simulink model "exploration"  (R2019a)
settings: Solver=FixedStepAuto  StartTime=0.0  StopTime=inf  FixedStep=0.001  RelTol=1e-3  EnableMultiTasking=on
settings Model: ExtModeTrigDuration=2  Creator=Dell  LastModifiedBy=Apple
settings OptimizationCC: EnhancedBackFolding=on  PassReuseOutputArgsAs=Individual arguments  MaxStackSize=64  OptimizeBlockOrder=speed  DifferentSizesBufferReuse=on  OptimizationCustomize=off
settings DebuggingCC: ParameterTunabilityLossMsg=error
settings HardwareCC: ProdBitPerInt=16  ProdBitPerPointer=16  ProdBitPerSizeT=16  ProdBitPerPtrDiffT=16  ProdLargestAtomicFloat=None  ProdWordSize=8  ProdHWDeviceType=Atmel->AVR  UseEmbeddedCoderFeatures=off
settings SFSimCC: MATLABDynamicMemAlloc=off
settings RTWCC: SystemTargetFile=ert.tlc  HardwareBoard=Arduino Mega 2560  TLCOptions=-aInlineSetEventsForThisBaseRateFcn=TLC_FALSE -aSuppressMultiTaskScheduler=TLC_FALSE -aRateBasedStepFcn=1  TemplateMakefile=ert_default_tmf  GenerateReport=on  Toolchain=Arduino AVR  BuildConfiguration=Faster Runs  IncludeHyperlinkInReport=on  LaunchReport=on  GenerateTraceInfo=on  GenerateTraceReport=on  GenerateTraceReportSl=on  GenerateTraceReportSf=on  GenerateTraceReportEml=on
settings CodeAppCC: ForceParamTrailComments=on  IgnoreCustomStorageClasses=off  OperatorAnnotations=on  SimulinkDataObjDesc=on  SFDataObjDesc=on  InsertBlockDesc=on
settings ERTTargetCC: SupportContinuousTime=on  SupportNonInlinedSFcns=on  SupportVariableSizeSignals=on  ExtModeStaticAllocSize=2048

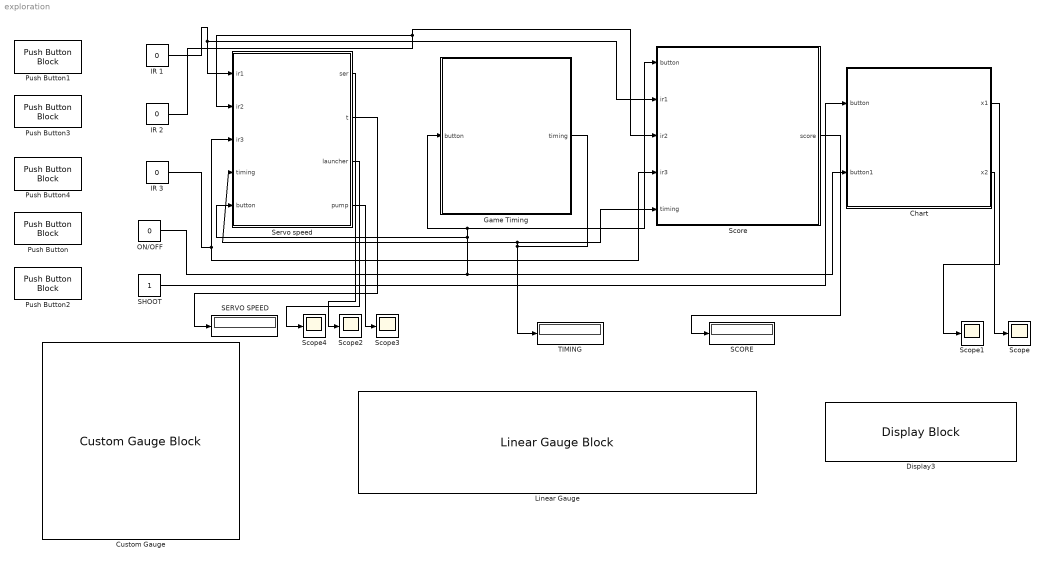
== system exploration ==
  Chart : Stateflow chart  BlockKeywords=__PRM__SERIALIZED__DATA__:Stateflow Chart,Stateflow Diagram  TreatAsAtomicUnit=on
  Custom Gauge : CustomGaugeBlock  NeedleImage=data:image/svg+xml;base64,PD94bWwgdmVyc2lvbj0iMS4wIiBlbmNvZGluZz0idXRmLTgiPz4KPCEtLSBHZW5lcmF0b3I6IEFkb2JlIElsbHVzdHJhdG9yIDE5LjIuMSwgU1ZHIEV4cG9ydCBQbHVnLUluIC4gU1ZHIFZlcnNpb246IDYuMDAgQnVpbGQgMCkgIC0tPgo8c3ZnIHZlcnNpb249IjEuMSIgeG1sbnM9Imh0dHA6Ly93d3cudzMub3JnLzIwMDAvc3ZnIiB4bWxuczp4bGluaz0iaHR0cDovL3d3dy53My5vcmcvMTk5OS94bGluayIgeD0iMHB4IiB5PSIwcHgiCgkgdmlld0JveD0iMCAwIDIwMCA1MCIgc3R5bGU9ImVuYWJsZS1iYWNrZ3JvdW5kOm5ldyAw ...(+9940 chars)  NeedleXPos=0.3802298124325669  NeedleYPos=0.48117305677424654  NeedleHeight=0.11602152693163792  NeedleWidth=0.1911368983686954  NeedleInitialRotation=-59.94322499147643  BackgroundImage=data:image/svg+xml;base64,PD94bWwgdmVyc2lvbj0iMS4wIiBlbmNvZGluZz0iVVRGLTgiIHN0YW5kYWxvbmU9Im5vIj8+CjwhLS0gR2VuZXJhdG9yOiBBZG9iZSBJbGx1c3RyYXRvciAxOS4yLjEsIFNWRyBFeHBvcnQgUGx1Zy1JbiAuIFNWRyBWZXJzaW9uOiA2LjAwIEJ1aWxkIDApICAtLT4KCjxzdmcKICAgeG1sbnM6ZGM9Imh0dHA6Ly9wdXJsLm9yZy9kYy9lbGVtZW50cy8xLjEvIgogICB4bWxuczpjYz0iaHR0cDovL2NyZWF0aXZlY29tbW9ucy5vcmcvbnMjIgogICB4bWxuczpyZGY9Imh0dHA6Ly93d3cudzMub3JnLzE5OTkvMDIvMjItcmRmLXN5bnRh ...(+9660 chars)  GaugeMax=30  GaugeArcDefined=true  GaugeArcRadius=0.1358563990074277  GaugeArcStrokeWidth=0.03972965542329953  GaugeArcRotation=240.5385250290321  GaugeArcRatio=0.8333333333333  GaugeArcTransparency=0  ValueArcColor=#1759b0  GaugeTickColor=#faf5c8  ScaleColorsJSON="[{\"Min\":0,\"Max\":9,\"Color\":[0.996078431372549,0.2,0.0392156862745098]},{\"Min\":9,\"Max\":21,\"Color\":[0.92941176470588238,0.69411764705882351,0.12549019607843137]},{\"Min\":21,\"Max\":30,\"Color\":[0.39215686274509803,0.83137254901960778,0.074509803921568626]}]"  fixedAspectRatio=on
  Display3 : DisplayBlock  LabelPosition=Hide  Format=short
  Game Timing : Stateflow chart  BlockKeywords=__PRM__SERIALIZED__DATA__:Stateflow Chart,Stateflow Diagram  TreatAsAtomicUnit=on
  IR 1 : Constant  Value=0  OutMin=[0]  OutMax=[1]
  IR 2 : Constant  Value=0  OutMin=[0]  OutMax=[1]
  IR 3 : Constant  Value=0  OutMin=[0]  OutMax=[1]
  Linear Gauge : LinearGaugeBlock  ScaleMin=10  ScaleMax=60
  ON/OFF : Constant  Value=0
  Push Button{,1..4} (5 alike) : PushButtonBlock
  SCORE : Display
  SERVO SPEED : Display
  SHOOT : Constant
  Scope{,1..4} (5 alike) : Scope
  Score : Stateflow chart  BlockKeywords=__PRM__SERIALIZED__DATA__:Stateflow Chart,Stateflow Diagram  TreatAsAtomicUnit=on
  Servo speed : Stateflow chart  BlockKeywords=__PRM__SERIALIZED__DATA__:Stateflow Chart,Stateflow Diagram  TreatAsAtomicUnit=on
  TIMING : Display
  wires:
  Servo speed/1(ser) -> Scope2/1
  IR 1/1 -> Score/2(ir1), Servo speed/1(ir1)
  Servo speed/2(t) -> SERVO SPEED/1
  IR 2/1 -> Score/3(ir2), Servo speed/2(ir2)
  IR 3/1 -> Score/4(ir3), Servo speed/3(ir3)
  ON/OFF/1 -> Chart/2(button1), Game Timing/1(button), Score/1(button), Servo speed/5(button)
  Game Timing/1(timing) -> TIMING/1, Score/5(timing), Servo speed/4(timing)
  Score/1(score) -> SCORE/1
  SHOOT/1 -> Chart/1(button)
  Chart/1(x1) -> Scope1/1
  Chart/2(x2) -> Scope/1
  Servo speed/3(launcher) -> Scope4/1
  Servo speed/4(pump) -> Scope3/1

== stateflow chart exploration/Game Timing ==
  state initialtime
    timing=30;
  state time1
    timing=timing;
  state time2
    timing=timing;
  time1 -> time2 [order 1] : [after(1,sec)&&timing>0]{timing = timing - 1}
  (default) -> initialtime
  initialtime -> time1 : [button==1]
  time1 -> initialtime [order 2] : [timing==0]
  time2 -> time1
  data: timing output; button input

== stateflow chart exploration/Score ==
  state scoring
    state score2
      score=score;
    state score3
      score=score;
    (default) -> score2
    score2 -> score3 [order 3] : [ir3==1]{score=score+20}
    score2 -> score3 [order 2] : [ir2==1]{score=score+15}
    score2 -> score3 [order 1] : [ir1==1]{score=score+10}
    score3 -> score2 : [after(250,msec)]
  state initialscore
  state initialscore1
    score=0;
  (default) -> initialscore
  initialscore -> initialscore1 : [button==1]
  initialscore1 -> scoring
  scoring -> initialscore : [timing==0]
  data: button input; ir1 input; ir2 input; ir3 input; timing input; score output

== stateflow chart exploration/Servo speed ==
  state main
    launcher=1;
    pump=1;
    state Servomotion
      state initial
        ser=10;
      state moving
        ser=ser;
      state Moving2
        ser=ser;
      (default) -> initial
      moving -> moving [order 1] : [after(t,msec)&&ser<170]{ser = ser + 1}
      initial -> moving
      Moving2 -> moving [order 2] : [ser==10]
      moving -> Moving2 [order 2] : [ser==170]
      Moving2 -> Moving2 [order 1] : [after(t,msec)&&ser>10]{ser = ser - 1}
    state dummy
    (default) -> Servomotion
    dummy -> Servomotion : [after(200,msec)]
    Servomotion -> dummy : [(ir1==1||ir2==1||ir3==1)&&t>10]{t=t-10}
  state initialtime
    t=60;
    launcher=0;
    pump=0;
  (default) -> initialtime
  initialtime -> main : [button==1]
  main -> initialtime : [timing==0]
  data: ser output; t output; ir1 input; ir2 input; ir3 input; timing input; launcher output; pump output; button input

== stateflow chart exploration/Chart ==
  state dcoff
    x1=0;
    x2=0;
  state dcon
    x1=1;
    x2=0;
  dcoff -> dcon : [button1==1&&button==1]
  (default) -> dcoff
  dcon -> dcoff : [after(0.299,sec)]
  data: button input; x1 output; x2 output; button1 input
